simulink model "simulationModel"  (R2017b)
settings: Solver=VariableStepAuto  StartTime=0.0  StopTime=Tmax  RelTol=1e-3
values from neighbouring files (symbols this model uses):
  A = A{1}    [TorquetoPRBS.m]    (also in simulationAnalysis.m = [I D K])
  fs = fs/df    (= 102.4)    [MS_static.m]    (also in Stiffness.m = 2048; TorquetoPRBS.m = 2048; simulationAnalysis.m)
settings Model: Creator=MoyaEstebanA  LastModifiedBy=MoyaEstebanA

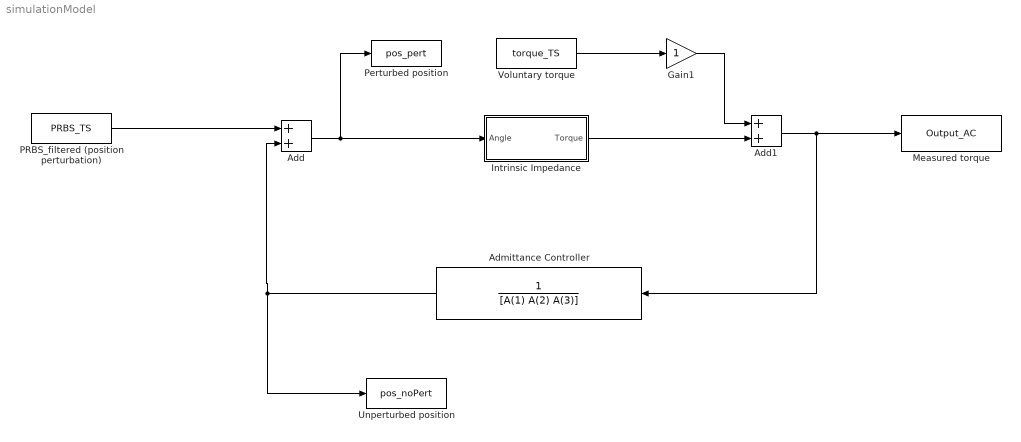
== system simulationModel ==
  Add : Sum
  Add1 : Sum
  Admittance Controller : TransferFcn  Denominator=[A(1) A(2) A(3)]
  Gain1 : Gain
  "Intrinsic Impedance " : Subsystem
  Measured torque : ToWorkspace  VariableName=Output_AC  SaveFormat=Timeseries  SampleTime=-1
  PRBS_filtered (position perturbation) : FromWorkspace  VariableName=PRBS_TS  SampleTime=1/fs
  Perturbed position : ToWorkspace  VariableName=pos_pert  SaveFormat=Timeseries  SampleTime=1/fs
  Unperturbed position : ToWorkspace  VariableName=pos_noPert  SaveFormat=Timeseries  SampleTime=1/fs
  Voluntary torque : FromWorkspace  VariableName=torque_TS  SampleTime=1/fs
  wires:
  PRBS_filtered (position perturbation)/1 -> Add/1
  Add/1 -> Perturbed position/1, "Intrinsic Impedance "/1(Angle)
  Add1/1 -> Admittance Controller/1, Measured torque/1
  Voluntary torque/1 -> Gain1/1
  "Intrinsic Impedance "/1(Torque) -> Add1/2
  Gain1/1 -> Add1/1
  Admittance Controller/1 -> Add/2, Unperturbed position/1

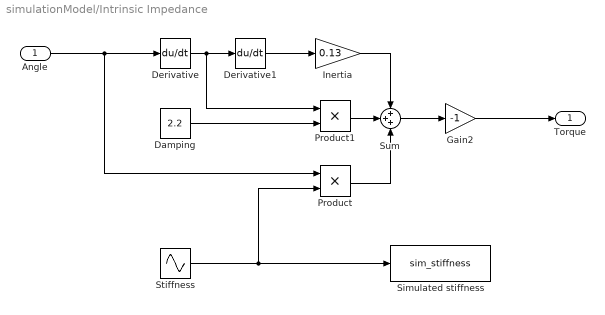
== system simulationModel/Intrinsic Impedance  ==
  Angle : Inport  SampleTime=1/fs
  Damping : Constant  Value=2.2  SampleTime=1/fs
  Derivative : Derivative
  Derivative1 : Derivative
  Gain2 : Gain  Gain=-1
  "Inertia " : Gain  Gain=0.13
  Product : Product  RndMeth=Zero
  Product1 : Product  RndMeth=Zero
  Simulated stiffness : ToWorkspace  VariableName=sim_stiffness  SaveFormat=Timeseries  SampleTime=1/fs
  Stiffness : Sin  Amplitude=10  Bias=30  Frequency=2*pi*0.5  SampleTime=1/fs
  Sum : Sum  Inputs=+++
  Torque : Outport  SampleTime=1/fs
  wires:
  Derivative/1 -> Derivative1/1, Product1/1
  Derivative1/1 -> "Inertia "/1
  "Inertia "/1 -> Sum/1
  Product1/1 -> Sum/2
  Product/1 -> Sum/3
  Sum/1 -> Gain2/1
  Gain2/1 -> Torque/1
  Damping/1 -> Product1/2
  Angle/1 -> Product/1, Derivative/1
  Stiffness/1 -> Simulated stiffness/1, Product/2
